simulink model "model"  (R2014b)
settings: Solver=FixedStepDiscrete  StartTime=0.0  StopTime=inf  FixedStep=Ts  RelTol=1e-3
InitFcn:
  | init;
StopFcn:
  | fini;
values from neighbouring files (symbols this model uses):
  d = 3    [init.m]
  k = 30    [init.m]
  plane_incl = 7.5 / 180 * pi    (= 0.1308996939)    [init.m]
libraries: WBCLibrary x9
settings Model: Creator=makaveli  LastModifiedBy=makaveli

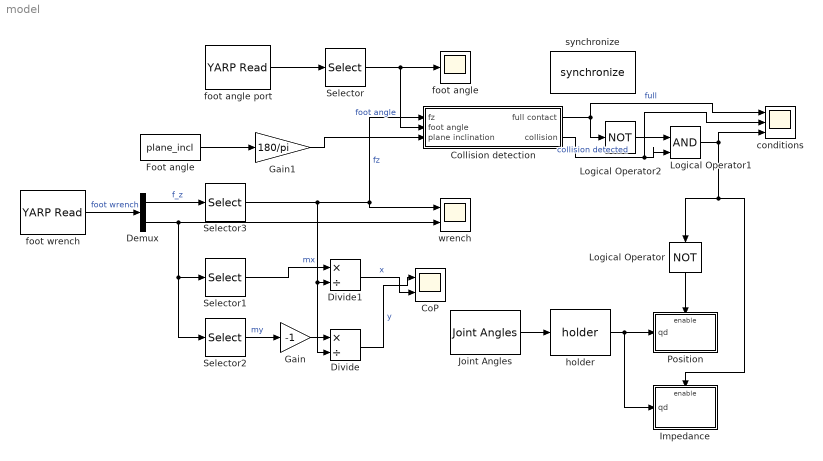
== system model ==
  CoP : Scope  NumInputPorts=2
      settings: TimeRange=10  YMin=-0.5~-5  YMax=0.5~5  SaveName=cop_left
  Collision detection : Subsystem
  Demux : Demux  Outputs=2
  Divide : Product  Inputs=*/
  Divide1 : Product  Inputs=*/
  Foot angle : Constant  Value=plane_incl
  Gain : Gain  Gain=-1
  Gain1 : Gain  Gain=180/pi
  Impedance : Subsystem
  Joint Angles : WBCLibrary/wholeBodyStates/Joint Angles  robotName=robotName  localName=localName
  Logical Operator : Logic  Operator=NOT  IconShape=distinctive  AllPortsSameDT=off  OutDataTypeStr=boolean
  Logical Operator1 : Logic  IconShape=distinctive  AllPortsSameDT=off  OutDataTypeStr=boolean
  Logical Operator2 : Logic  Operator=NOT  IconShape=distinctive  AllPortsSameDT=off  OutDataTypeStr=boolean
  Position : Subsystem
  Selector : Selector  InputPortWidth=12  Indices=[2]
  Selector1 : Selector  InputPortWidth=3  Indices=[1]
  Selector2 : Selector  InputPortWidth=3  Indices=[2]
  Selector3 : Selector  InputPortWidth=3  Indices=[3]
  conditions : Scope  NumInputPorts=3
      settings: YMin=-5~-5~-5  YMax=5~5~5  SaveName=conditions
  foot angle : Scope
      settings: SaveName=foot_angle
  foot angle port : WBCLibrary/Utilities/YARP Read  portName='/icubGazeboSim/left_foot/inertial'  signalSize=12  blocking=off  timestamp=off  autoconnect=on
  foot wrench : WBCLibrary/Utilities/YARP Read  portName='/icubGazeboSim/left_foot/analog:o'  signalSize=6  blocking=off  timestamp=off  autoconnect=on
  "holder " : WBCLibrary/Utilities/holder 
  synchronize : WBCLibrary/Utilities/synchronize  rate=Ts  scaleFactor=1
  wrench : Scope  NumInputPorts=2
      settings: ShowLegends=on  YMin=-5~-5  YMax=5~5  SaveName=wrench
  wires:
  foot angle port/1 -> Selector/1
  Selector/1 -> Collision detection/2(foot angle), foot angle/1  "foot angle"
  foot wrench/1 -> Demux/1  "foot wrench"
  Demux/2 -> wrench/2, Selector2/1, Selector1/1
  Demux/1 -> Selector3/1  "f_z"
  Joint Angles/1 -> "holder "/1
  "holder "/1 -> Impedance/1(qd), Position/1("qd ")
  Logical Operator/1 -> Position/Enable
  Foot angle/1 -> Gain1/1
  Collision detection/1(full contact) -> Logical Operator2/1, conditions/1  "full"
  Collision detection/2(collision) -> conditions/2, Logical Operator1/2  "collision detected"
  Logical Operator2/1 -> Logical Operator1/1
  Logical Operator1/1 -> Logical Operator/1, Impedance/Enable, conditions/3
  Selector3/1 -> Divide/2, Divide1/2, Collision detection/1(fz), wrench/1  "fz"
  Selector2/1 -> Gain/1  "my"
  Gain/1 -> Divide/1
  Divide1/1 -> CoP/2  "x"
  Divide/1 -> CoP/1  "y"
  Selector1/1 -> Divide1/1  "mx"
  Gain1/1 -> Collision detection/3(plane inclination)

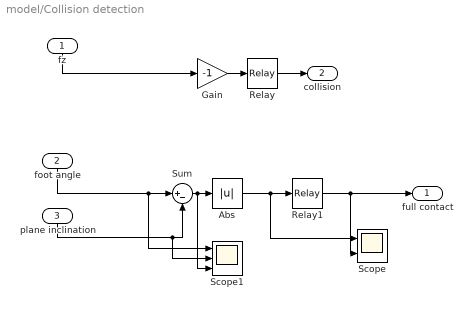
== system model/Collision detection ==
  fz : Inport
  foot angle : Inport  Port=2
  plane inclination : Inport  Port=3
  Abs : Abs
  Gain : Gain  Gain=-1
  Relay : Relay  OnSwitchValue=500  OffSwitchValue=-500
  Relay1 : Relay  OnSwitchValue=1  OffSwitchValue=0.5  OnOutputValue=0  OffOutputValue=1
  Scope : Scope  NumInputPorts=2
      settings: YMin=-5~-5  YMax=5~5  SaveName=ScopeData3
  Scope1 : Scope  NumInputPorts=3
      settings: YMin=-5~-5~-5  YMax=5~5~5  SaveName=ScopeData4
  Sum : Sum  Inputs=|+-
  full contact : Outport
  collision : Outport  Port=2
  wires:
  fz/1 -> Gain/1
  Relay/1 -> collision/1
  Gain/1 -> Relay/1
  foot angle/1 -> Scope1/1, Sum/1
  plane inclination/1 -> Scope1/2, Sum/2
  Sum/1 -> Scope1/3, Abs/1
  Relay1/1 -> full contact/1, Scope/2
  Abs/1 -> Relay1/1, Scope/1

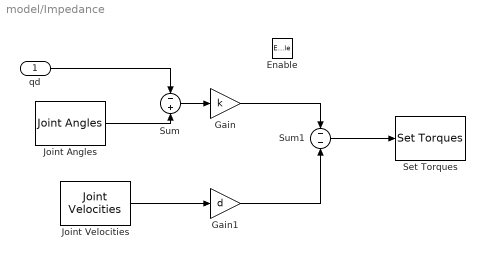
== system model/Impedance ==
  qd : Inport
  Enable : EnablePort
  Gain : Gain  Gain=k
  Gain1 : Gain  Gain=d
  Joint Angles : WBCLibrary/wholeBodyStates/Joint Angles  robotName=robotName  localName=localName
  Joint Velocities : WBCLibrary/wholeBodyStates/Joint Velocities  robotName=robotName  localName=localName
  Set Torques : WBCLibrary/wholeBodyActuators/Set Torques  val=6  robotName=robotName  localName=localName
  Sum : Sum  Inputs=-+
  Sum1 : Sum  Inputs=--
  wires:
  qd/1 -> Sum/1
  Joint Angles/1 -> Sum/2
  Sum/1 -> Gain/1
  Joint Velocities/1 -> Gain1/1
  Sum1/1 -> Set Torques/1
  Gain/1 -> Sum1/1
  Gain1/1 -> Sum1/2

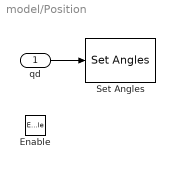
== system model/Position ==
  "qd " : Inport
  Enable : EnablePort
  Set Angles : WBCLibrary/wholeBodyActuators/Set Angles  val=5  robotName=robotName  localName=localName
  wires:
  "qd "/1 -> Set Angles/1
